simulink model "lab1_system4"  (R2024a)
settings: Solver=VariableStepAuto  StartTime=0.0  StopTime=10.0  RelTol=1e-3
settings Model: Creator=alexivanov  LastModifiedBy=alexivanov

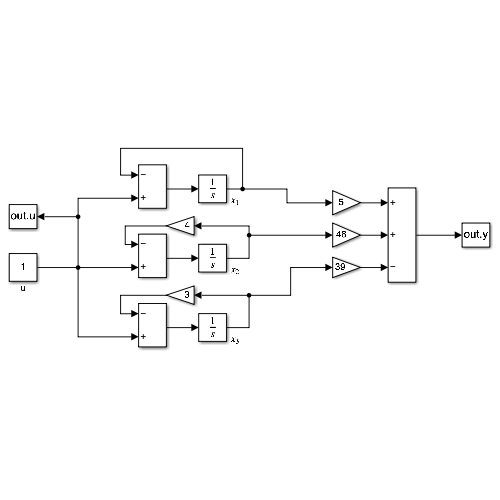
[thumbnail: Simulink's stored preview of the top-level diagram]
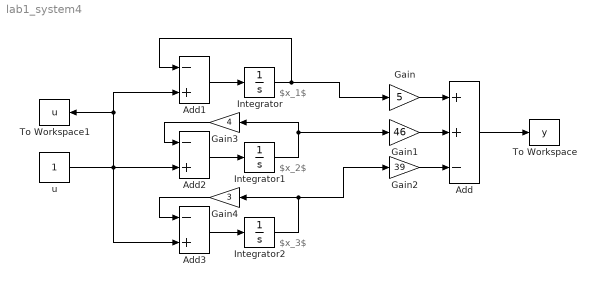
== system lab1_system4 ==
  note: $x_1$
  note: $x_2$
  note: $x_3$
  Add : Sum  Inputs=++-
  Add1 : Sum  Inputs=-+
  Add2 : Sum  Inputs=-+
  Add3 : Sum  Inputs=-+
  Gain : Gain  Gain=5
  Gain1 : Gain  Gain=46
  Gain2 : Gain  Gain=39
  Gain3 : Gain  Gain=4
  Gain4 : Gain  Gain=3
  Integrator : Integrator
  Integrator1 : Integrator
  Integrator2 : Integrator
  To Workspace : ToWorkspace  VariableName=y  SaveFormat=Timeseries  SampleTime=-1
  To Workspace1 : ToWorkspace  VariableName=u  SaveFormat=Timeseries  SampleTime=-1
  u : Constant  SampleTime=0
  wires:
  Gain/1 -> Add/1
  Gain1/1 -> Add/2
  Gain2/1 -> Add/3
  Add/1 -> To Workspace/1
  Integrator/1 -> Add1/1, Gain/1
  u/1 -> Add3/2, Add1/2, To Workspace1/1, Add2/2
  Add1/1 -> Integrator/1
  Integrator1/1 -> Gain1/1, Gain3/1
  Add2/1 -> Integrator1/1
  Gain3/1 -> Add2/1
  Gain4/1 -> Add3/1
  Integrator2/1 -> Gain2/1, Gain4/1
  Add3/1 -> Integrator2/1
